simulink model "Electrical_Vehicle"  (R2015a)
settings: Solver=ode45  StartTime=0.0  StopTime=10.0  RelTol=1e-3
libraries: sdl_lib x7, fl_lib x4, elec_lib x3, nesl_utility x2
settings Model: Creator=Galib  LastModifiedBy=Galib

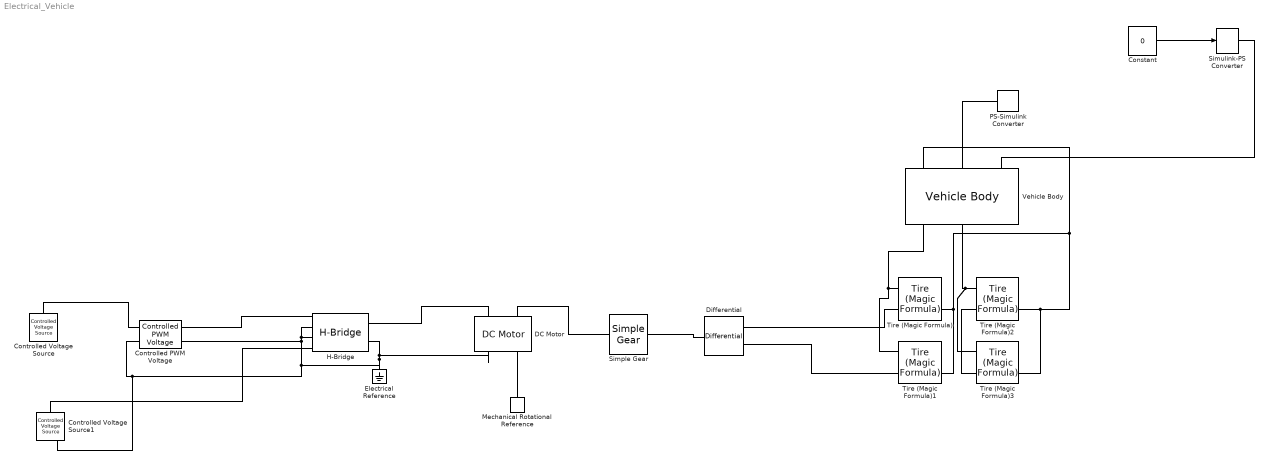
== system Electrical_Vehicle ==
  Constant : Constant  Value=0  VectorParams1D=off  SampleTime=-1
  Controlled PWM Voltage : elec_lib/Actuators & Drivers/Drivers/Controlled PWM Voltage  F=1000 Hz  TD=0 s  pulse_width_offset=0 s  Vmin=0 V  Vmax=0 V  Vm=1 V  pwm_or_av=2  event_type=1  sample_time=1e-6 s
  Controlled Voltage Source : fl_lib/Electrical/Electrical Sources/Controlled Voltage Source
  Controlled Voltage Source1 : fl_lib/Electrical/Electrical Sources/Controlled Voltage Source
  DC Motor : elec_lib/Actuators & Drivers/Rotational Actuators/DC Motor  parameterization=3  Ra=3.9 Ohm  La=1.2e-5 H  emf_or_torque=1  Kv=7.2e-5 V/rpm  Ki=6.876e-4 N*m/A  T_stall=2.4e-4 N*m  w_max=15000 rpm  w_rated=12000 rpm  P_rated=35000 W  V_rated=50 V  J=0.01 g*cm^2  lam_param=1  lam=0 N*m/(rad/s)  i_noload=0 A  V_i_noload=1.5 V  speed0=0 rpm  alpha=0.00393 1/K  Tmeas=25 C  thermal_mass=100 J/K  initial_temperature=25 C
  Differential : sdl_lib/Gears/Differential  driveshaft_location=2  cd_ratio=4  friction_model=1  efficiency=[ 0.85 0.92 ]  mu_visc=[ 0 0 ] N*m/(rad/s)  w_thr=[ 0.01 0.01 ] rad/s  temperature_TLU=[ 280 300 320 ] K  efficiency_ss_TLU=[ 0.95 0.9 0.85 ]  efficiency_cd_TLU=[ 0.95 0.9 0.85 ]  thermal_mass=50 J/K  T_init=300 K
  Electrical Reference : fl_lib/Electrical/Electrical Elements/Electrical Reference
  H-Bridge : elec_lib/Actuators & Drivers/Drivers/H-Bridge  Venable=2.5 V  Vmax=5.0 V  Vreverse=2.5 V  Vbrake=2.5 V  Vm=12 V  pwm_or_av=2  discontinuous=1  freewheeling_mode=1  freewheeling_mode_disc=1  Ron=0.1 Ohm  Don=0.05 Ohm  Rload=10 Ohm  Lload=1e-5 H  F=10 kHz  thermal_mass=100 J/K  initial_temperature=298.15 K  Ron2=0.1 Ohm  Don2=0.05 Ohm  Tmeas=298.15 K  Tmeas2=398.15 K
  Mechanical Rotational Reference : fl_lib/Mechanical/Rotational Elements/Mechanical Rotational Reference
  PS-Simulink Converter : nesl_utility/PS-Simulink Converter  PhysicalDomain=network_engine_domain  SubClassName=ps_output  LeftPortType=input  RightPortType=output  PseudoPeriodic=off  Frequencies=[]  Unit=km/hr  AffineConversion=off
  Simple Gear : sdl_lib/Gears/Simple Gear  ratio=3  rotation_direction=2  friction_model=1  T_noload=0.1 N*m  T_nom=5 N*m  efficiency_nom=0.8  efficiency=0.8  mu_visc=[ 0 0 ] N*m/(rad/s)  w_thr=0.01 rad/s  temperature_TLU=[ 280 300 320 ] K  load_TLU=[ 1 5 10 ] N*m  efficiency_TLU=[ 0.95 0.9 0.85 ]  efficiency_TLU2=[ 0.85 0.8 0.75; 0.95 0.9 0.85; 0.85 0.8 0.7 ]  thermal_mass=50 J/K  T_init=300 K
  Simulink-PS Converter : nesl_utility/Simulink-PS Converter  PhysicalDomain=network_engine_domain  SubClassName=ps_input  LeftPortType=input  RightPortType=output  PseudoPeriodic=off  Frequencies=[]  NoiseDistribution=none  NoiseParameters=[]  Unit=1  AffineConversion=off  InputFiltering=off  SimscapeFilterOrder=1  InputFilterTimeConstant=0.001  UdotUserProvided=1
  Tire (Magic Formula){,1..3} (4 alike) : sdl_lib/Tires & Vehicles/Tire (Magic Formula)  parameterization=1  F_z1=3e+3 N  F_x1=3.5e+3 N  kappa1=10  B_m=10  C_m=1.9  D_m=1  E_m=0.97  fz0=4e+3 N  p_Cx=1.685  p_Dx=[ 1.21 -0.037 ]  p_Ex=[ 0.344 0.095 -0.02 0 ]  p_Kx=[ 21.51 -0.163 0.245 ]  p_Hx=[ -0.002 0.002 ]  p_Vx=[ 0 0 ]  v_tr_thr=0.1 m/s  r_e=0.3 m  model_compliance=0  stiffness=1e+6 N/m  damping=1000 N/(m/s)  model_inertia=0  inertia=1 kg*m^2  initial_velocity=0 rad/s  model_resistance=1  resistance_model=1  coeff=0.013  p_tire=250e3 Pa  alpha=-0.003  beta=0.97  coeff_a=84e-4  coeff_b=6.2e-4 s/m  coeff_c=1.6e-4 s^2/m^2  v_thr=1e-3 m/s
  Vehicle Body : sdl_lib/Tires & Vehicles/Vehicle Body  mass=1000 kg  n_w=2  x_f=1.4 m  x_r=1.6 m  y_c=0.5 m  area=2.5 m^2  Cd=0.4  v0=0 m/s  g=9.81 m/s^2  rho=1.18 kg/m^3
  wires:
  Constant/1 -> Simulink-PS Converter/1
  connections:
  PS-Simulink Converter/LConn1 -- Vehicle Body/LConn2
  Simulink-PS Converter/RConn1 -- Vehicle Body/LConn3
  Vehicle Body/RConn1 -- Tire (Magic Formula)1/LConn1 -- Tire (Magic Formula)/LConn1
  Tire (Magic Formula)2/LConn1 -- Vehicle Body/RConn2 -- Tire (Magic Formula)3/LConn1
  Tire (Magic Formula)2/LConn2 -- Tire (Magic Formula)3/LConn2
  Tire (Magic Formula)2/RConn2 -- Tire (Magic Formula)/RConn2 -- Tire (Magic Formula)1/RConn2 -- Vehicle Body/LConn1 -- Tire (Magic Formula)3/RConn2
  Differential/RConn2 -- Tire (Magic Formula)/LConn2
  Differential/RConn1 -- Tire (Magic Formula)1/LConn2
  Simple Gear/RConn1 -- Differential/LConn1
  Simple Gear/LConn1 -- DC Motor/LConn2
  DC Motor/RConn2 -- Mechanical Rotational Reference/LConn1
  H-Bridge/RConn1 -- DC Motor/LConn1
  H-Bridge/RConn2 -- DC Motor/RConn1 -- Controlled Voltage Source1/RConn2 -- Controlled PWM Voltage/LConn2 -- Controlled PWM Voltage/RConn2 -- H-Bridge/LConn2 -- H-Bridge/LConn3 -- Electrical Reference/LConn1
  Controlled PWM Voltage/RConn1 -- H-Bridge/LConn1
  Controlled Voltage Source/LConn1 -- Controlled PWM Voltage/LConn1
  Controlled Voltage Source1/LConn1 -- H-Bridge/LConn4
